simulink model "WT_MPPT_SCOPES_FINAL"  (R2025a)
settings: Solver=VariableStepAuto  StartTime=0.0  StopTime=11  RelTol=1e-3
settings Model: Creator=hero  LastModifiedBy=hero

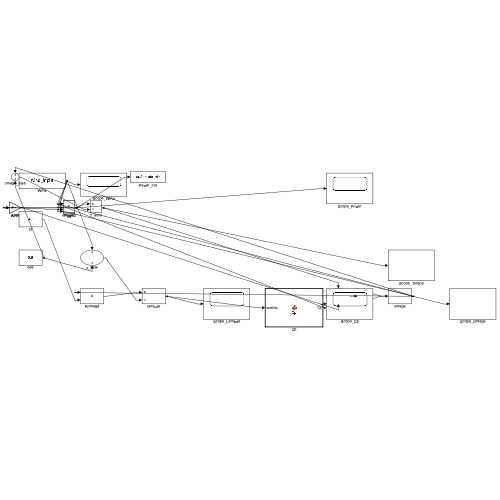
[thumbnail: Simulink's stored preview of the top-level diagram]
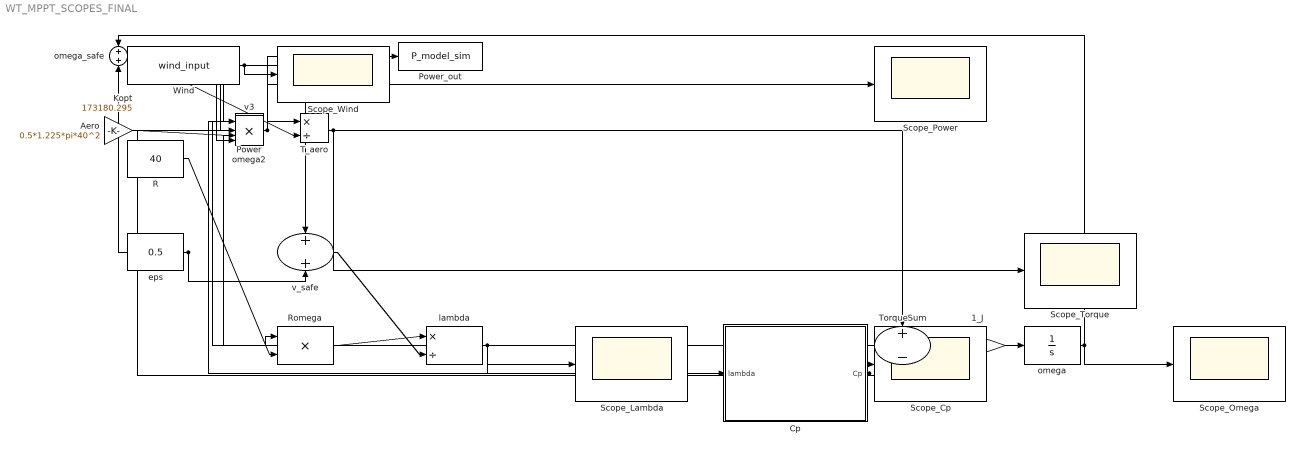
== system WT_MPPT_SCOPES_FINAL ==
  1_J : Gain  Gain=1/500000
  Aero : Gain  Gain=0.5*1.225*pi*40^2
  Cp : MATLAB Function  TreatAsAtomicUnit=on
  Kopt : Gain  Gain=173180.295
  Power : Product
  Power_out : ToWorkspace  VariableName=P_model_sim  SampleTime=-1
  R : Constant  Value=40
  Romega : Product
  Scope_Cp : Scope
  Scope_Lambda : Scope
  Scope_Omega : Scope
  Scope_Power : Scope
  Scope_Torque : Scope
  Scope_Wind : Scope
  T_aero : Product  Inputs=*/
  TorqueSum : Sum  Inputs=+-
  Wind : FromWorkspace  VariableName=wind_input
  eps : Constant  Value=0.5
  lambda : Product  Inputs=*/
  omega : Integrator  InitialCondition=1
  omega2 : Product
  omega_safe : Sum
  v3 : Product  Inputs=3
  v_safe : Sum
  wires:
  Wind/1 -> Scope_Wind/1, v_safe/1, v3/1, v3/2, v3/3
  omega/1 -> Scope_Omega/1, Romega/1, omega_safe/1, omega2/1, omega2/2
  lambda/1 -> Scope_Lambda/1, Cp/1(lambda)
  Cp/1(Cp) -> Scope_Cp/1, Power/1
  R/1 -> Romega/2
  eps/1 -> v_safe/2, omega_safe/2
  Romega/1 -> lambda/1
  v_safe/1 -> lambda/2
  v3/1 -> Aero/1
  Aero/1 -> Power/2
  Power/1 -> Scope_Power/1, Power_out/1, T_aero/1
  omega_safe/1 -> T_aero/2
  T_aero/1 -> Scope_Torque/1, TorqueSum/1
  omega2/1 -> Kopt/1
  Kopt/1 -> TorqueSum/2
  TorqueSum/1 -> 1_J/1
  1_J/1 -> omega/1

== matlab function WT_MPPT_SCOPES_FINAL/Cp ==
  data: lambda input; Cp output
function Cp = Cp(lambda)
lambda = max(lambda,0.1);
lambda = min(lambda,12);
lambda_i = 1/(1/(lambda+0.08)-0.035);
Cp = 0.22*((116/lambda_i)-5)*exp(-12.5/lambda_i);
Cp = max(min(Cp,0.48),0);
end
